simulink model "model_matematyczny_2019b"  (R2019b)
settings: Solver=VariableStepAuto  StartTime=0.0  StopTime=30  RelTol=1e-3
libraries: eeStairGenerator x1
settings Model: Creator=Admin  LastModifiedBy=dawid
settings DebuggingCC: UnconnectedInputMsg=none  UnconnectedOutputMsg=none  UnconnectedLineMsg=none  SFMachineParentedDataDiag=error

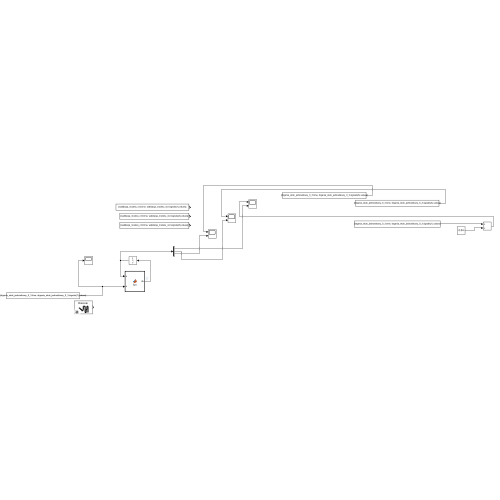
[thumbnail: Simulink's stored preview of the top-level diagram]
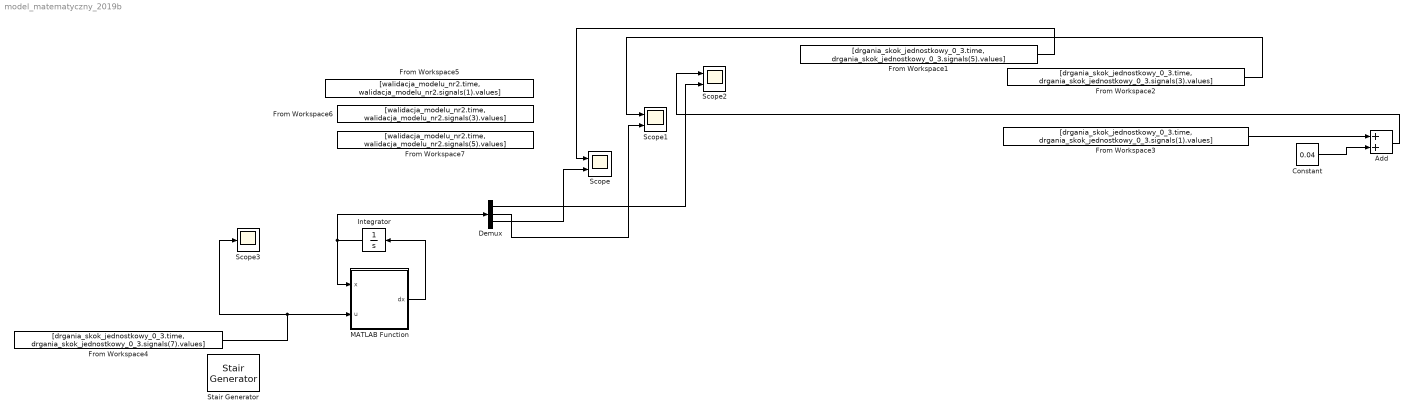
== system model_matematyczny_2019b ==
  Add : Sum
  Constant : Constant  Value=0.04
  Demux : Demux  Outputs=3
  From Workspace1 : FromWorkspace  VariableName=[drgania_skok_jednostkowy_0_3.time, drgania_skok_jednostkowy_0_3.signals(5).values]
  From Workspace2 : FromWorkspace  VariableName=[drgania_skok_jednostkowy_0_3.time, drgania_skok_jednostkowy_0_3.signals(3).values]
  From Workspace3 : FromWorkspace  VariableName=[drgania_skok_jednostkowy_0_3.time, drgania_skok_jednostkowy_0_3.signals(1).values]
  From Workspace4 : FromWorkspace  VariableName=[drgania_skok_jednostkowy_0_3.time, drgania_skok_jednostkowy_0_3.signals(7).values]
  From Workspace5 : FromWorkspace  VariableName=[walidacja_modelu_nr2.time, walidacja_modelu_nr2.signals(1).values]
  From Workspace6 : FromWorkspace  VariableName=[walidacja_modelu_nr2.time, walidacja_modelu_nr2.signals(3).values]
  From Workspace7 : FromWorkspace  VariableName=[walidacja_modelu_nr2.time, walidacja_modelu_nr2.signals(5).values]
  Integrator : Integrator  InitialCondition=[0, 0, 0]
  MATLAB Function : MATLAB Function  TreatAsAtomicUnit=on
  Scope : Scope  NumInputPorts=2
  Scope1 : Scope  NumInputPorts=2
  Scope2 : Scope  NumInputPorts=2
  Scope3 : Scope
  Stair Generator : eeStairGenerator/Stair Generator  LabelModeActiveChoice=Discrete  TimeInput=[0, 4, 9, 13, 14, 20, 23, 26, 29]  AmplitudeInput=[0.4, 0, -0.4, 0, 1, -1, 0, 1, -1]  SampleTime=0.01  RepeatPattern=off  OutDataTypeStr=double
      settings: SourceProductBaseCode=PS
  wires:
  MATLAB Function/1(dx) -> Integrator/1
  Integrator/1 -> MATLAB Function/1(x), Demux/1
  Demux/2 -> Scope1/2
  Demux/3 -> Scope/2
  Demux/1 -> Scope2/2
  From Workspace3/1 -> Add/1
  Constant/1 -> Add/2
  From Workspace1/1 -> Scope/1
  From Workspace2/1 -> Scope1/1
  Add/1 -> Scope2/1
  From Workspace4/1 -> Scope3/1, MATLAB Function/2(u)

== matlab function model_matematyczny_2019b/MATLAB Function ==
  data: x input; u input; dx output
% function dx = fcn(x, u)
% 
% %dane wyidentyfikowane
% MgL = 0.1064;
% g = 9.81;
% kt = 0.027; % NmA
% R = 0.4; %Ohmy
% 
% mi_phi = 0.000082; 
% % mi_phi = 1.566850664740816e-04;
% % mi_theta = 0.0290; %zostało wyznaczone z drgań swobodnych 
% mi_theta = 0.0290;
% 
% G = 488.7;
% J = 0.0283; %kg*m^2
% 
% %wspołczynnik a:
% % a = 0.0023;
% % b = -0.0022;
% p = [0.002321260244060,-0.002210724041962];
% dx = [0 0 0];
% dx(1) = x(2); % pochodna polozenia
% dx(2) = (1/J)*(MgL * sin(x(1)) - mi_theta * x(2) + (((kt * kt)/R) + mi_phi) * x(3) - kt*u/R); % pochodna predkosci obrotowe belki
% dx(3) = G * (u - polyval(p, x(3))); %pochodna predkosci smigla 
% 
% end


function dx = fcn(x, u)

%dane wyidentyfikowane
MgL = 0.1064;
g = 9.81;
kt = 0.027; % NmA
ke = 0.025;
R = 2.4; %Ohmy

% mi_phi = 0.000644785835713765; 
mi_phi = 0.0000882;
% mi_theta = 0.00000132; %zostało wyznaczone z drgań swobodnych 
mi_theta = 0.0290;

G = 488.648;
% J = 0.0185; %kg*m^2
J = 0.0219;
%wspołczynnik a:
% a = 0.0023;
% b = -0.0022;
p = [0.002314296507890,-8.816367649105842e-04];
dx = [0 0 0];
dx(1) = x(2); % pochodna polozenia
% dx(2) = (1/J)*(-MgL * sin(x(1)) - mi_theta * x(2) + (((kt * ke)/R) + mi_phi) * x(3) - kt*u/R); % pochodna predkosci obrotowe belki
dx(2) = (1/J)*(-MgL * sin(x(1)) - mi_theta * x(2) - (kt * (u*12 - ke * x(3)) / R) + mi_phi * x(3));
dx(3) = G * (u - polyval(p, x(3))); %pochodna predkosci smigla 

end
